simulink model "sim_espaco_de_estados"  (R2016a)
settings: Solver=ode14x  StartTime=0.0  StopTime=25  FixedStep=0.001  RelTol=1e-3
InitFcn:
  | clear all;
  | Kpx = 10;
  | Kix = 25;
  | Kpy = 10;
  | Kiy = 25;
  | Kvphi = 3;
  | Kpphi = 2.25;
  | 
  | Kem = 0.0059;
  | Kti = 0.0059;
  | Vd = 5.4;
  | R = 1.71;
  | r = 0.072;
  | eta = 0.83;
  | N = 19;
  | 
  | Jw = 8.1e-4;
  | 
  | mi = 0.25;
  | b = .1;
  | 
  | Ts = 0.0001;
values from neighbouring files (symbols this model uses):
  g = 9.8    [resultados_velocidade_linear_constante.mat]
  M = 1.83    [resultados_velocidade_linear_constante.mat]
libraries: simulink x1
settings Model: Creator=Pichau  LastModifiedBy=Pichau

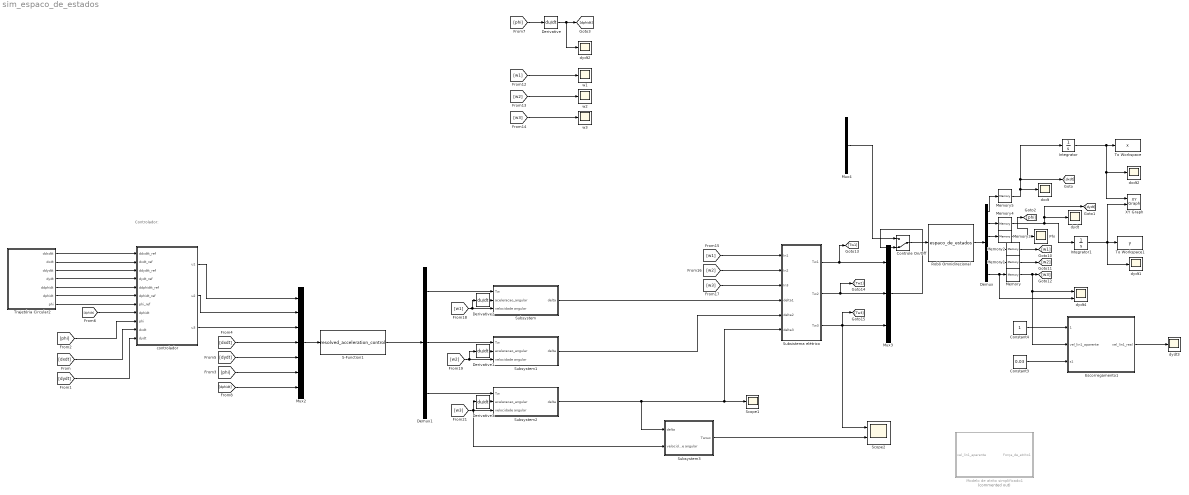
== system sim_espaco_de_estados ==
  note: Controlador:
  Constant3 : Constant  Value=0.03
  Constant4 : Constant
  Controle On/Off : ManualSwitch  CurrentSetting=0
  Demux : Demux  Outputs=6
  Demux1 : Demux  Outputs=3
  Derivative{,1..3} (4 alike) : Derivative
  Escorregamento1 : Subsystem
  Integrator : Integrator  InitialCondition=0.3
  Integrator1 : Integrator
  Memory{,1..2,4..5} (5 alike) : Memory
  Memory3 : Memory  X0=pi/2
  Modelo de atrito simplificado1 : Subsystem  Commented=on
  Mux2 : Mux  Inputs=7
  Mux3 : Mux  Inputs=3
  Mux4 : Mux  Inputs=3
  Phi : Scope
  Robô Omnidirecional : S-Function  FunctionName=espaco_de_estados  Parameters=r,m,Jw,J,L  SFunctionDeploymentMode=off  EnableBusSupport=off  mask{r=0.072, m=1.71, Jw=8.1e-4, J=2.125, L=0.09}
      mask prompts: r "r (m)"; m "m (Kg)"; Jw "Jw (Kg*m^2)"; J "J (Kg*m^2)"; L "L (m)"
      mask Display: image(imread('Robot_omnidirectional_drive.png'));
  S-Function1 : S-Function  FunctionName=resolved_acceleration_control  Parameters=r,L,m,J,Jw  SFunctionDeploymentMode=off  EnableBusSupport=off  mask{r=0.072, L=0.09, m=1.71, J=2.125, Jw=8.1e-4}
  Scope1 : Scope
  Scope2 : Scope  NumInputPorts=2
  Subsistema elétrico : Subsystem
  Subsystem : Subsystem
  Subsystem1 : Subsystem
  Subsystem2 : Subsystem
  Subsystem3 : Subsystem
  To Workspace : ToWorkspace  VariableName=x  SaveFormat=Timeseries  SampleTime=-1
  To Workspace1 : ToWorkspace  VariableName=y  SaveFormat=Timeseries  SampleTime=-1
  Trajetória Circular2 : Subsystem
  XY Graph : simulink/Sinks/XY Graph  xmin=-1  xmax=1  ymin=-1  ymax=1  st=-1
  controlador : Subsystem
  dxdt : Scope
  dxdt2 : Scope
  dydt{,1..3} (4 alike) : Scope
  dydt4 : Scope  NumInputPorts=2
  w1 : Scope
  w2 : Scope
  w3 : Scope
  wires:
  Robô Omnidirecional/1 -> Demux/1
  Integrator1/1 -> XY Graph/2, To Workspace1/1, dydt1/1
  Integrator/1 -> XY Graph/1, dxdt2/1, To Workspace/1
  Trajetória Circular2/2(dxdt) -> controlador/2(dxdt_ref)
  Trajetória Circular2/6(dphidt) -> controlador/6(dphidt_ref)
  Trajetória Circular2/1(ddxdtt) -> controlador/1(ddxdtt_ref)
  Trajetória Circular2/4(dydt) -> controlador/4(dydt_ref)
  Trajetória Circular2/3(ddydtt) -> controlador/3(ddydtt_ref)
  Trajetória Circular2/7(phi) -> controlador/7(phi_ref)
  Trajetória Circular2/5(ddphidt) -> controlador/5(ddphidtt_ref)
  controlador/1(u1) -> Mux2/1
  controlador/2(u2) -> Mux2/2
  controlador/3(u3) -> Mux2/3
  [dxdt] -> controlador/10(dxdt)
  [dydt] -> controlador/11(dydt)
  [phi] -> controlador/9(phi)
  Mux2/1 -> S-Function1/1
  [dphidt] -> controlador/8(dphidt)
  Derivative/1 -> dydt2/1, [dphidt]
  S-Function1/1 -> Demux1/1
  Mux3/1 -> Controle On/Off/2
  Controle On/Off/1 -> Robô Omnidirecional/1
  [w3] -> w3/1
  [w2] -> w2/1
  [w1] -> w1/1
  Demux/1 -> Memory5/1
  Demux/2 -> Memory4/1
  Demux/3 -> Memory3/1
  [phi] -> Derivative/1
  [dxdt] -> Mux2/4
  [dydt] -> Mux2/5
  [phi] -> Mux2/6
  [dphidt] -> Mux2/7
  Demux/4 -> Memory2/1
  Demux/5 -> Memory1/1
  Demux/6 -> dydt4/2, Memory/1
  [w1] -> Subsistema elétrico/1(In1)
  [w2] -> Subsistema elétrico/2(In2)
  [w3] -> Subsistema elétrico/3(In3)
  Subsistema elétrico/3(Tw3) -> Scope2/1, [Tw3], Mux3/3
  Subsistema elétrico/2(Tw2) -> [Tw2], Mux3/2
  Subsistema elétrico/1(Tw1) -> [Tw1], Mux3/1
  Mux4/1 -> Controle On/Off/1
  Demux1/1 -> Subsystem/1(Tw)
  Demux1/2 -> Subsystem1/1(Tw)
  Demux1/3 -> Subsystem2/1(Tw)
  Subsystem1/1(delta) -> Subsistema elétrico/5(delta2)
  Subsystem/1(delta) -> Subsistema elétrico/4(delta1)
  [w1] -> Derivative2/1, Subsystem/3(velocidade angular)
  [w2] -> Derivative1/1, Subsystem1/3(velocidade angular)
  [w3] -> Subsystem3/2(velocidade angular), Derivative3/1, Subsystem2/3(velocidade angular)
  Derivative1/1 -> Subsystem1/2(aceleracao_angular)
  Derivative2/1 -> Subsystem/2(aceleracao_angular)
  Derivative3/1 -> Subsystem2/2(aceleracao_angular)
  Constant3/1 -> Escorregamento1/3(s1)
  Constant4/1 -> Escorregamento1/1(1)
  Escorregamento1/1("vel_lin1_real ") -> dydt3/1
  Memory/1 -> Escorregamento1/2("vel_lin1_aparente "), dydt4/1, [w3]
  Memory1/1 -> [w2]
  Memory2/1 -> [w1]
  Memory3/1 -> Phi/1, [phi]
  Memory4/1 -> Integrator1/1, [dydt], dydt/1
  Memory5/1 -> [dxdt], Integrator/1, dxdt/1
  Subsystem2/1(delta) -> Subsystem3/1(delta), Subsistema elétrico/6(delta3), Scope1/1
  Subsystem3/1(Twww) -> Scope2/2

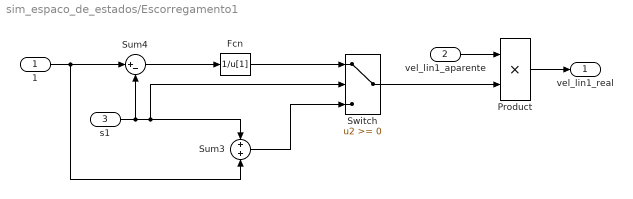
== system sim_espaco_de_estados/Escorregamento1 ==
  1 : Inport
  "vel_lin1_aparente " : Inport  Port=2
  s1 : Inport  Port=3
  Fcn : Fcn  Expr=1/u[1]
  Product : Product  RndMeth=Zero
  Sum3 : Sum  Inputs=+|+
  Sum4 : Sum  Inputs=|+-
  Switch : Switch
  "vel_lin1_real " : Outport
  wires:
  s1/1 -> Switch/2, Sum3/1, Sum4/2
  1/1 -> Sum3/2, Sum4/1
  Sum4/1 -> Fcn/1
  Fcn/1 -> Switch/1
  Sum3/1 -> Switch/3
  Switch/1 -> Product/2
  "vel_lin1_aparente "/1 -> Product/1
  Product/1 -> "vel_lin1_real "/1

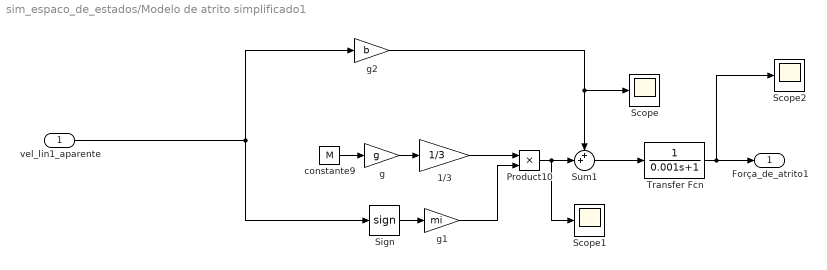
== system sim_espaco_de_estados/Modelo de atrito simplificado1 ==
  vel_lin1_aparente : Inport
  1/3 : Gain  Gain=1/3
  Product10 : Product  RndMeth=Zero
  Scope : Scope
  Scope1 : Scope
  Scope2 : Scope
  Sign : Signum
  Sum1 : Sum  Inputs=++|
  Transfer Fcn : TransferFcn  Denominator=[0.001 1]
  constante9 : Constant  Value=M
  g : Gain  Gain=g
  g1 : Gain  Gain=mi
  g2 : Gain  Gain=b
  Força_de_atrito1 : Outport
  wires:
  Transfer Fcn/1 -> Força_de_atrito1/1, Scope2/1
  g2/1 -> Scope/1, Sum1/1
  Sum1/1 -> Transfer Fcn/1
  Sign/1 -> g1/1
  vel_lin1_aparente/1 -> Sign/1, g2/1
  Product10/1 -> Sum1/2, Scope1/1
  g1/1 -> Product10/2
  1/3/1 -> Product10/1
  g/1 -> 1/3/1
  constante9/1 -> g/1

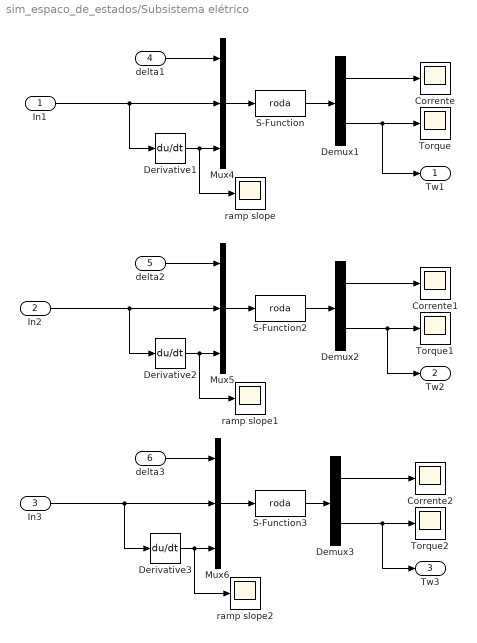
== system sim_espaco_de_estados/Subsistema elétrico ==
  In1 : Inport
  In2 : Inport  Port=2
  In3 : Inport  Port=3
  delta1 : Inport  Port=4
  delta2 : Inport  Port=5
  delta3 : Inport  Port=6
  Corrente : Scope
  Corrente1 : Scope
  Corrente2 : Scope
  Demux1 : Demux  Outputs=2
  Demux2 : Demux  Outputs=2
  Demux3 : Demux  Outputs=2
  Derivative1 : Derivative
  Derivative2 : Derivative
  Derivative3 : Derivative
  Mux4 : Mux  Inputs=3
  Mux5 : Mux  Inputs=3
  Mux6 : Mux  Inputs=3
  S-Function : S-Function  FunctionName=roda  Parameters=Vd,Vsat,deltaVd,L,Kem,R,Kti,Jm,eta,N  SFunctionDeploymentMode=off  EnableBusSupport=off  mask{Vd=6, Vsat=0.3, deltaVd=0, L=0.00011, Kem=0.0059, R=1.71, Kti=0.0059, Jm=3.88e-7, eta=0.83, N=19}
  S-Function2 : S-Function  FunctionName=roda  Parameters=Vd,Vsat,deltaVd,L,Kem,R,Kti,Jm,eta,N  SFunctionDeploymentMode=off  EnableBusSupport=off  mask{Vd=6, Vsat=0.3, deltaVd=0, L=0.00011, Kem=0.0059, R=1.71, Kti=0.0059, Jm=3.88e-7, eta=0.83, N=19}
  S-Function3 : S-Function  FunctionName=roda  Parameters=Vd,Vsat,deltaVd,L,Kem,R,Kti,Jm,eta,N  SFunctionDeploymentMode=off  EnableBusSupport=off  mask{Vd=6, Vsat=0.3, deltaVd=0, L=0.00011, Kem=0.0059, R=1.71, Kti=0.0059, Jm=3.88e-7, eta=0.83, N=19}
  Torque : Scope
  Torque1 : Scope
  Torque2 : Scope
  ramp slope : Scope
  ramp slope1 : Scope
  ramp slope2 : Scope
  Tw1 : Outport
  Tw2 : Outport  Port=2
  Tw3 : Outport  Port=3
  wires:
  Demux3/1 -> Corrente2/1
  Mux6/1 -> S-Function3/1
  Derivative3/1 -> ramp slope2/1, Mux6/3
  Demux3/2 -> Tw3/1, Torque2/1
  In3/1 -> Mux6/2, Derivative3/1
  S-Function3/1 -> Demux3/1
  delta2/1 -> Mux5/1
  delta3/1 -> Mux6/1
  Mux5/1 -> S-Function2/1
  In2/1 -> Derivative2/1, Mux5/2
  S-Function2/1 -> Demux2/1
  Demux2/1 -> Corrente1/1
  Demux2/2 -> Tw2/1, Torque1/1
  Derivative2/1 -> Mux5/3, ramp slope1/1
  Derivative1/1 -> ramp slope/1, Mux4/3
  In1/1 -> Mux4/2, Derivative1/1
  Demux1/2 -> Tw1/1, Torque/1
  Mux4/1 -> S-Function/1
  S-Function/1 -> Demux1/1
  delta1/1 -> Mux4/1
  Demux1/1 -> Corrente/1

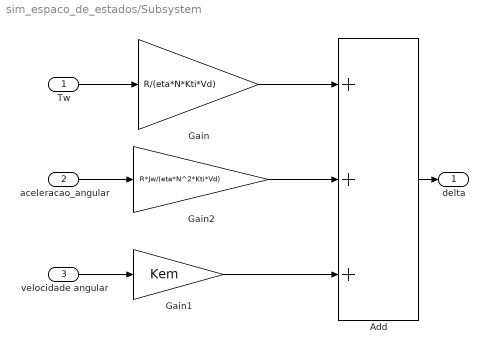
== system sim_espaco_de_estados/Subsystem ==
  Tw : Inport
  aceleracao_angular : Inport  Port=2
  velocidade angular : Inport  Port=3
  Add : Sum  Inputs=+++
  Gain : Gain  Gain=R/(eta*N*Kti*Vd)
  Gain1 : Gain  Gain=Kem
  Gain2 : Gain  Gain=R*Jw/(eta*N^2*Kti*Vd)
  delta : Outport
  wires:
  aceleracao_angular/1 -> Gain2/1
  velocidade angular/1 -> Gain1/1
  Add/1 -> delta/1
  Tw/1 -> Gain/1
  Gain1/1 -> Add/3
  Gain/1 -> Add/1
  Gain2/1 -> Add/2

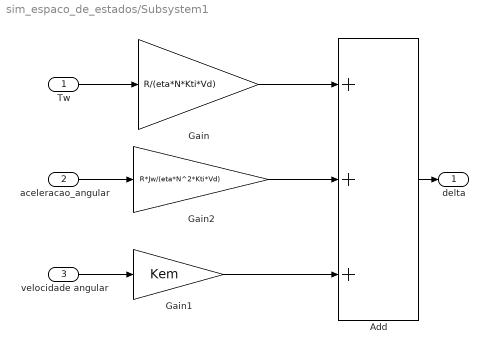
== system sim_espaco_de_estados/Subsystem1 ==
  Tw : Inport
  aceleracao_angular : Inport  Port=2
  velocidade angular : Inport  Port=3
  Add : Sum  Inputs=+++
  Gain : Gain  Gain=R/(eta*N*Kti*Vd)
  Gain1 : Gain  Gain=Kem
  Gain2 : Gain  Gain=R*Jw/(eta*N^2*Kti*Vd)
  delta : Outport
  wires:
  Gain2/1 -> Add/2
  Gain/1 -> Add/1
  Gain1/1 -> Add/3
  Tw/1 -> Gain/1
  Add/1 -> delta/1
  velocidade angular/1 -> Gain1/1
  aceleracao_angular/1 -> Gain2/1

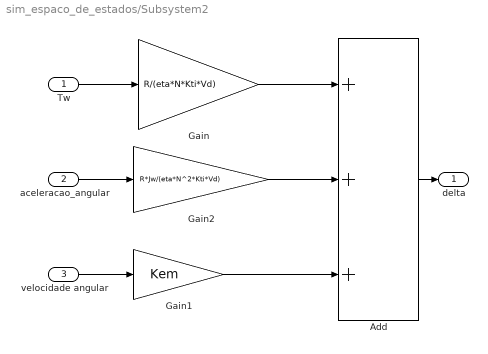
== system sim_espaco_de_estados/Subsystem2 ==
  Tw : Inport
  aceleracao_angular : Inport  Port=2
  velocidade angular : Inport  Port=3
  Add : Sum  Inputs=+++
  Gain : Gain  Gain=R/(eta*N*Kti*Vd)
  Gain1 : Gain  Gain=Kem
  Gain2 : Gain  Gain=R*Jw/(eta*N^2*Kti*Vd)
  delta : Outport
  wires:
  aceleracao_angular/1 -> Gain2/1
  velocidade angular/1 -> Gain1/1
  Add/1 -> delta/1
  Tw/1 -> Gain/1
  Gain1/1 -> Add/3
  Gain/1 -> Add/1
  Gain2/1 -> Add/2

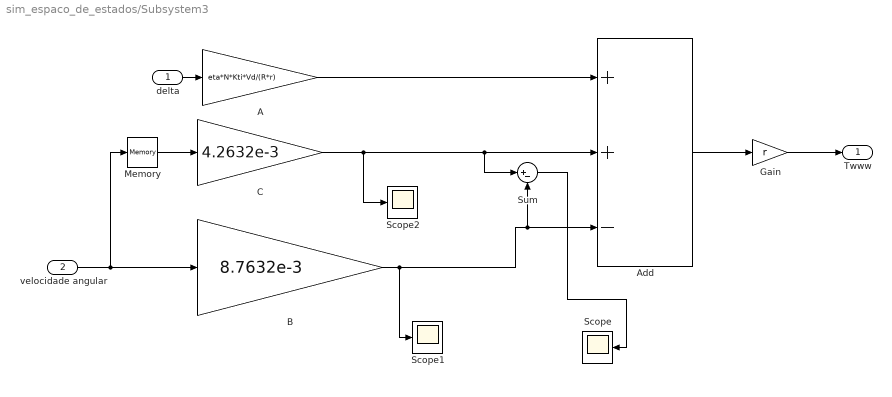
== system sim_espaco_de_estados/Subsystem3 ==
  delta : Inport
  velocidade angular : Inport  Port=2
  A : Gain  Gain=eta*N*Kti*Vd/(R*r)
  Add : Sum  Inputs=++-
  B : Gain  Gain=8.7632e-3
  C : Gain  Gain=4.2632e-3
  Gain : Gain  Gain=r
  Memory : Memory
  Scope : Scope
  Scope1 : Scope
  Scope2 : Scope
  Sum : Sum  Inputs=|+-
  Twww : Outport
  wires:
  Add/1 -> Gain/1
  delta/1 -> A/1
  velocidade angular/1 -> Memory/1, B/1
  A/1 -> Add/1
  Memory/1 -> C/1
  Gain/1 -> Twww/1
  C/1 -> Scope2/1, Sum/1, Add/2
  Sum/1 -> Scope/1
  B/1 -> Scope1/1, Add/3, Sum/2

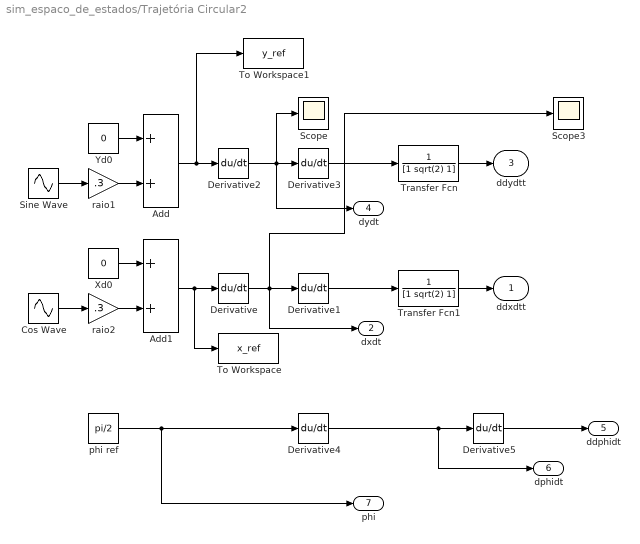
== system sim_espaco_de_estados/Trajetória Circular2 ==
  Add : Sum
  Add1 : Sum
  Cos Wave : Sin  Frequency=0.3  Phase=pi/2  SampleTime=0
  Derivative{,1..5} (6 alike) : Derivative
  Scope : Scope
  Scope3 : Scope
  Sine Wave : Sin  Frequency=0.3  SampleTime=0
  To Workspace : ToWorkspace  VariableName=x_ref  SaveFormat=Timeseries  SampleTime=-1
  To Workspace1 : ToWorkspace  VariableName=y_ref  SaveFormat=Timeseries  SampleTime=-1
  Transfer Fcn : TransferFcn  Denominator=[1 sqrt(2) 1]
  Transfer Fcn1 : TransferFcn  Denominator=[1 sqrt(2) 1]
  Xd0 : Constant  Value=0
  Yd0 : Constant  Value=0
  phi ref : Constant  Value=pi/2
  raio1 : Gain  Gain=.3
  raio2 : Gain  Gain=.3
  ddxdtt : Outport
  dxdt : Outport  Port=2
  ddydtt : Outport  Port=3
  dydt : Outport  Port=4
  ddphidt : Outport  Port=5
  dphidt : Outport  Port=6
  phi : Outport  Port=7
  wires:
  Transfer Fcn1/1 -> ddxdtt/1
  Transfer Fcn/1 -> ddydtt/1
  Derivative5/1 -> ddphidt/1
  Derivative1/1 -> Transfer Fcn1/1
  Derivative3/1 -> Transfer Fcn/1
  Derivative2/1 -> Derivative3/1, Scope/1, dydt/1
  Derivative/1 -> Scope3/1, Derivative1/1, dxdt/1
  Sine Wave/1 -> raio1/1
  raio1/1 -> Add/2
  Add/1 -> To Workspace1/1, Derivative2/1
  Add1/1 -> To Workspace/1, Derivative/1
  raio2/1 -> Add1/2
  Cos Wave/1 -> raio2/1
  Xd0/1 -> Add1/1
  Yd0/1 -> Add/1
  phi ref/1 -> Derivative4/1, phi/1
  Derivative4/1 -> Derivative5/1, dphidt/1

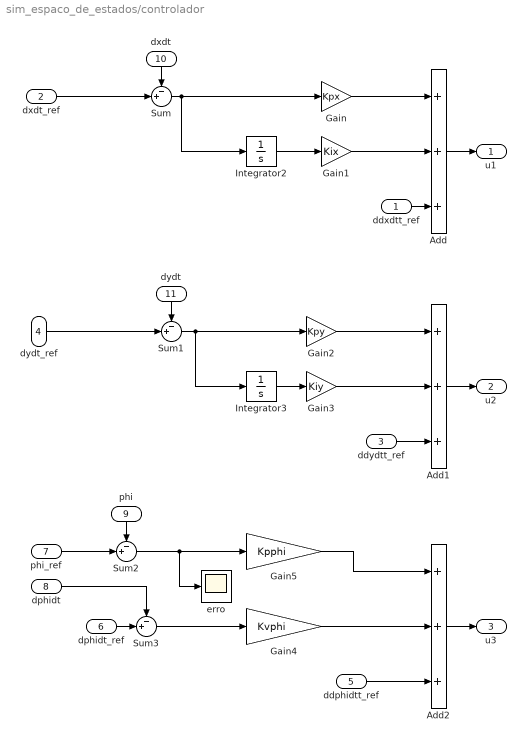
== system sim_espaco_de_estados/controlador ==
  ddxdtt_ref : Inport
  dxdt_ref : Inport  Port=2
  ddydtt_ref : Inport  Port=3
  dydt_ref : Inport  Port=4
  ddphidtt_ref : Inport  Port=5
  dphidt_ref : Inport  Port=6
  phi_ref : Inport  Port=7
  dphidt : Inport  Port=8
  phi : Inport  Port=9
  dxdt : Inport  Port=10
  dydt : Inport  Port=11
  Add : Sum  Inputs=+++
  Add1 : Sum  Inputs=+++
  Add2 : Sum  Inputs=+++
  Gain : Gain  Gain=Kpx
  Gain1 : Gain  Gain=Kix
  Gain2 : Gain  Gain=Kpy
  Gain3 : Gain  Gain=Kiy
  Gain4 : Gain  Gain=Kvphi
  Gain5 : Gain  Gain=Kpphi
  Integrator2 : Integrator
  Integrator3 : Integrator
  Sum{,1..3} (4 alike) : Sum  Inputs=-+|
  erro : Scope
  u1 : Outport
  u2 : Outport  Port=2
  u3 : Outport  Port=3
  wires:
  Sum2/1 -> Gain5/1, erro/1
  Sum1/1 -> Gain2/1, Integrator3/1
  Gain1/1 -> Add/2
  Integrator2/1 -> Gain1/1
  dydt_ref/1 -> Sum1/2
  Add/1 -> u1/1
  Gain2/1 -> Add1/1
  Integrator3/1 -> Gain3/1
  dphidt/1 -> Sum3/1
  Gain4/1 -> Add2/2
  Sum/1 -> Gain/1, Integrator2/1
  Gain3/1 -> Add1/2
  Gain5/1 -> Add2/1
  Sum3/1 -> Gain4/1
  ddphidtt_ref/1 -> Add2/3
  ddydtt_ref/1 -> Add1/3
  Add1/1 -> u2/1
  ddxdtt_ref/1 -> Add/3
  phi/1 -> Sum2/1
  Add2/1 -> u3/1
  dxdt_ref/1 -> Sum/2
  dxdt/1 -> Sum/1
  phi_ref/1 -> Sum2/2
  Gain/1 -> Add/1
  dydt/1 -> Sum1/1
  dphidt_ref/1 -> Sum3/2
